simulink model "system_id_new"  (R2023a)
settings: Solver=ode1  StartTime=0.0  StopTime=Sim_time+10  FixedStep=0.002  RelTol=1e-3  EnableMultiTasking=on
values from neighbouring files (symbols this model uses):
  dt = 0.002    [repeated_daqne.m]    (also in test.m)
  frequency = 10.^[f_low:(f_up - f_low)/N_d:f_up-(f_up - f_low)/N_d]'    [repeated_daqne.m]    (also in test.m)
  gain = gain_tuning*rand(size(frequency))    [repeated_daqne.m]    (also in test.m)
  phase = rand(size(frequency))    [repeated_daqne.m]    (also in test.m)
undefined symbols (not defined in the file or in its folder): HIL
libraries: quarc_library x5, slpidlib x1
settings Model: SimulationMode=external  Creator=kentaroohki  LastModifiedBy=Flexible4
settings SolverCC: AlgebraicLoopSolver=TrustRegion  PositivePriorityOrder=on
settings DataIOCC: SaveOperatingPoint=on  SaveFormat=Structure  SaveOutput=off  SignalLogging=off  DSMLogging=off  InspectSignalLogs=on  SaveTime=off  ReturnWorkspaceOutputs=off
settings DebuggingCC: UnconnectedInputMsg=warning  UnconnectedOutputMsg=warning  UnconnectedLineMsg=warning  ArithmeticOperatorsInVariantConditions=warning
settings ModelReferenceCC: EnableRefExpFcnMdlSchedulingChecks=on
settings SFSimCC: SimUseLocalCustomCode=off  CustomCodeUndefinedFunction=UseInterfaceOnly
settings RTWCC: Description=QUARC Win64 Target Using Toolchain  SystemTargetFile=quarc_win64.tlc  TemplateMakefile=quarc_default_tmf  RTWUseLocalCustomCode=off  Toolchain=QUARC win64 | nmake (64-bit Windows)  BuildConfiguration=Faster Runs
settings STFCustomTargetCC: SystemTargetFile=quarc_win64.tlc
settings GRTTargetCC: ParMdlRefBuildCompliant=off  CompOptLevelCompliant=off  CombineOutputUpdateFcns=off  MatFileLogging=off  CPPClassGenCompliant=off  GRTInterface=on  ExtMode=on  ExtModeMexFile=quarc_comm

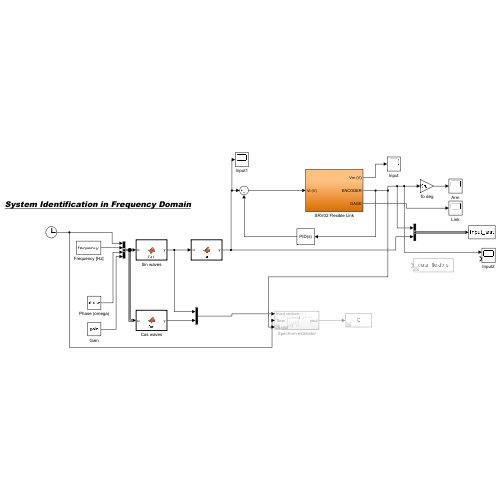
[thumbnail: Simulink's stored preview of the top-level diagram]
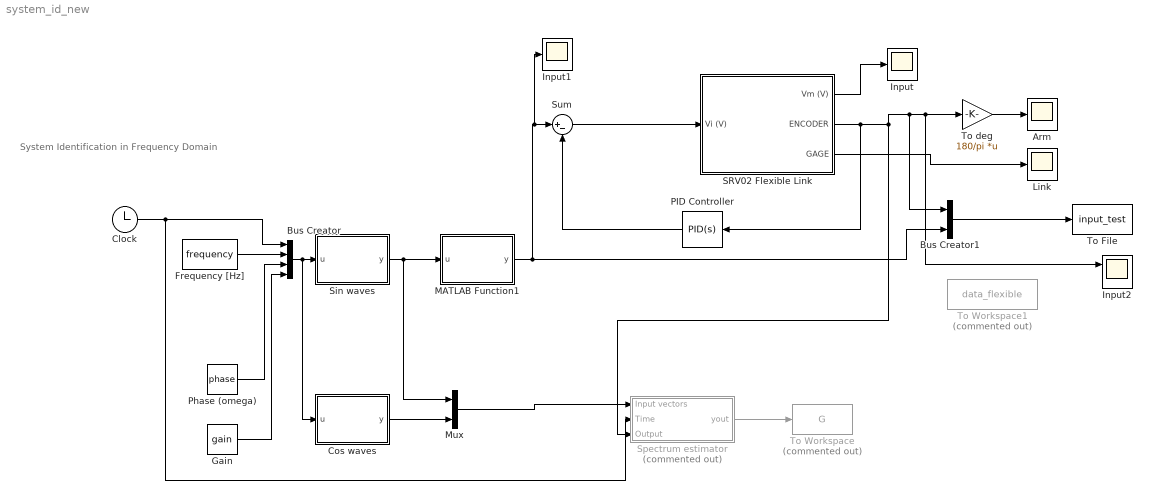
== system system_id_new ==
  note: System Identification in Frequency Domain
  Arm : Scope
  Bus Creator : BusCreator  Inputs=4
  Bus Creator1 : BusCreator  Inputs=2
  Clock : Clock
  Cos waves : MATLAB Function  TreatAsAtomicUnit=on
  Frequency [Hz] : Constant  Value=frequency  VectorParams1D=off
  Gain : Constant  Value=gain  VectorParams1D=off
  Input : Scope
  Input1 : Scope
  Input2 : Scope  NumInputPorts=2
  Link : Scope
  MATLAB Function1 : MATLAB Function  TreatAsAtomicUnit=on
  Mux : Mux  Inputs=2
  PID Controller : slpidlib/PID Controller  Controller=PID  Form=Parallel  TimeDomain=Continuous-time  UseExternalTs=off  SampleTime=-1  IntegratorMethod=Forward Euler  FilterMethod=Forward Euler  ControllerParametersSource=internal  P=1.65  I=0  UseKiTs=off  D=0  N=100  UseFilter=on  TunerSelectOption=Transfer Function Based (PID Tuner App)  InitialConditionSource=internal  InitialConditionForIntegrator=0  InitialConditionForFilter=0  DifferentiatorICPrevScaledInput=0  ExternalReset=none  TrackingMode=off  Kt=1  LimitOutput=off  SatLimitsSource=internal  UpperSaturationLimit=inf  LowerSaturationLimit=-inf  LinearizeAsGain=on  AntiWindupMode=none  Kb=1  LimitIntegrator=off  UpperIntegratorSaturationLimit=inf  LowerIntegratorSaturationLimit=-inf  POutMin=[]  POutMax=[]  IOutMin=[]  IOutMax=[]  DOutMin=[]  DOutMax=[]  NOutMin=[]  NOutMax=[]  SumOutMin=[]  SumOutMax=[]  SaturationOutMin=[]  SaturationOutMax=[]  PParamMin=[]  PParamMax=[]  IParamMin=[]  IParamMax=[]  DParamMin=[]  DParamMax=[]  NParamMin=[]  NParamMax=[]  KbParamMin=[]  KbParamMax=[]  KtParamMin=[]  KtParamMax=[]  KbOutMin=[]  KbOutMax=[]  KtOutMin=[]  KtOutMax=[]  IntegratorOutMin=[]  IntegratorOutMax=[]  FilterOutMin=[]  FilterOutMax=[]  SumI1OutMin=[]  SumI1OutMax=[]  SumI2OutMin=[]  SumI2OutMax=[]  SumI3OutMin=[]  SumI3OutMax=[]  SumI4OutMin=[]  SumI4OutMax=[]  SumDOutMin=[]  SumDOutMax=[]  DifferentiatorOutMin=[]  DifferentiatorOutMax=[]  FilterDiffOutCoefMin=[]  FilterDiffOutCoefMax=[]  ReciprocalOutMin=[]  ReciprocalOutMax=[]  SumDenOutMin=[]  SumDenOutMax=[]  SumNumOutMin=[]  SumNumOutMax=[]  DivideOutMin=[]  DivideOutMax=[]  UdiffTsProdOutMin=[]  UdiffTsProdOutMax=[]  NTsProdOutMin=[]  NTsProdOutMax=[]  UintegralTsProdOutMin=[]  UintegralTsProdOutMax=[]  UngainTsProdOutMin=[]  UngainTsProdOutMax=[]  ClampingZeroOutDataTypeStr=Inherit: Inherit via back propagation  ClampingZeroOutMin=[]  ClampingZeroOutMax=[]  FilterDenConstantOutDataTypeStr=Inherit: Inherit via back propagation  FilterDenConstantOutMin=[]  FilterDenConstantOutMax=[]  PCopyOutDataTypeStr=Inherit: Inherit via back propagation  PCopyOutMin=[]  PCopyOutMax=[]  NCopyOutDataTypeStr=Inherit: Inherit via back propagation  NCopyOutMin=[]  NCopyOutMax=[]  IntegratorContinuousStateAttributes=''  IntegratorStateMustResolveToSignalObject=off  IntegratorRTWStateStorageClass=Auto  FilterContinuousStateAttributes=''  FilterStateMustResolveToSignalObject=off  FilterRTWStateStorageClass=Auto  ParallelPVariant=InternalParameters  IdealPVariant=Disabled  IVariant=InternalParameters  DVariant=InternalParameters  IntegratorVariant=Continuous  SatVariant=Disabled  AWVariant=Passthrough  PCopyVariant=Disabled  TRVariant=Disabled  FdbkBlocksVariant=Forward  IdealPFdbkVariant=Disabled  SatFdbkVariant=Disabled  DerivativeFilterVariant=ContFilter  NVariant=InternalParameters  NCopyVariant=Disabled  FilterICVariant=InternalICsFilter  IntegratorICVariant=InternalICs  ExternalResetVariant=Disabled  TRSumVariant=Passthrough  SumFdbkVariant=Disabled  SumVariant=Sum_PID  TsampFilterVariant=InternalTs  TsampNgainVariant=Passthrough  TsampIntegralVariant=Disabled_SignalSpec  ExternalSaturationOutDataTypeStr=Inherit: Same as second input
  Phase (omega) : Constant  Value=phase  VectorParams1D=off
  SRV02 Flexible Link : Subsystem
  Sin waves : MATLAB Function  TreatAsAtomicUnit=on
  Spectrum estimator : Subsystem  Commented=on
  Sum : Sum  Inputs=|+-
  To File : ToFile  Filename=input_test  MatrixName=output
  To Workspace : ToWorkspace  Commented=on  VariableName=G  SampleTime=dt
      settings: Decimation=decim
  To Workspace1 : ToWorkspace  Commented=on  VariableName=data_flexible  SampleTime=-1
      settings: Save2DSignal=2-D array (concatenate along first dimension)
  To deg : Gain  Gain=180/pi  Multiplication=Matrix(K*u)
  wires:
  SRV02 Flexible Link/3(GAGE) -> Link/1
  Clock/1 -> Spectrum estimator/2(Time), Bus Creator/1
  Frequency [Hz]/1 -> Bus Creator/2
  Phase (omega)/1 -> Bus Creator/3
  Bus Creator/1 -> Cos waves/1(u), Sin waves/1(u)
  Gain/1 -> Bus Creator/4
  Sin waves/1(y) -> Mux/1, MATLAB Function1/1(u)
  MATLAB Function1/1(y) -> Bus Creator1/2, Input1/1, Sum/1
  Spectrum estimator/1(yout) -> To Workspace/1
  Cos waves/1(y) -> Mux/2
  Mux/1 -> Spectrum estimator/1(Input vectors)
  To deg/1 -> Arm/1
  SRV02 Flexible Link/1(Vm (V)) -> Input/1
  SRV02 Flexible Link/2(ENCODER) -> PID Controller/1, Bus Creator1/1, Input2/1, To deg/1, Spectrum estimator/3(Output)
  Sum/1 -> SRV02 Flexible Link/1(Vi (V))
  PID Controller/1 -> Sum/2
  Bus Creator1/1 -> To File/1

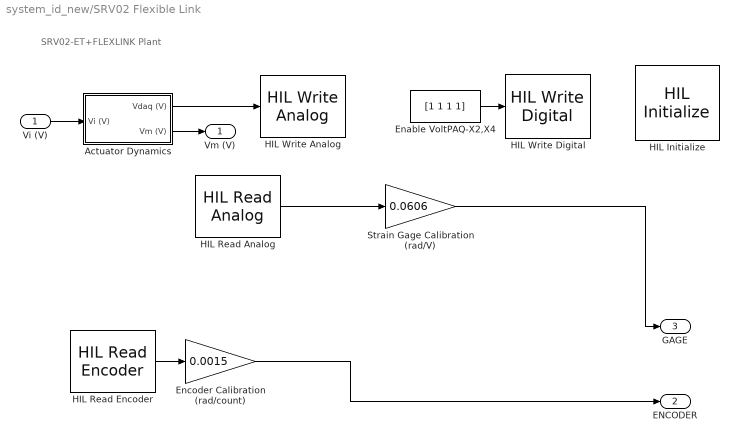
== system system_id_new/SRV02 Flexible Link ==
  note: SRV02-ET+FLEXLINK Plant
  Vi (V) : Inport
  Actuator Dynamics : Subsystem
  Enable VoltPAQ-X2,X4 : Constant  Value=[1 1 1 1]
  Encoder Calibration (rad/count) : Gain  Gain=0.0015  SaturateOnIntegerOverflow=on  OutDataTypeStr=Inherit: Same as input  ParamDataTypeStr=Inherit: Same as input
  HIL Initialize : quarc_library/Data Acquisition/Generic/Configuration/HIL Initialize  object_name=HIL-1  board_type=q2_usb  board_number=0  board_options=d0=digital;d1=digital;led=auto;update_rate=normal  exclusive=off  active=off  hardware_clocks=[0:2]  clock_modes=[]  initial_clock_frequencies=[]  set_clock_params_at_start=off  set_clock_params_at_switch_in=off  set_clock_frequencies_at_start=off  set_clock_frequencies_at_switch_in=off  analog_input_channels=[0:1]  analog_input_configurations=[]  analog_input_maximums=10  analog_input_minimums=-10  set_analog_input_params_at_start=on  set_analog_input_params_at_switch_in=off  analog_output_channels=[0:1]  analog_output_maximums=10  analog_output_minimums=-10  initial_analog_outputs=[0]  final_analog_outputs=[0]  watchdog_analog_outputs=0  set_analog_output_params_at_start=on  set_analog_output_params_at_switch_in=off  set_analog_outputs_at_start=on  set_analog_outputs_at_switch_in=off  set_analog_outputs_at_terminate=on  set_analog_outputs_at_switch_out=off  set_analog_outputs_on_watchdog=off  digital_input_channels=[]  digital_output_channels=[0:7]  digital_output_configuration=[]  initial_digital_outputs=[0]  final_digital_outputs=[0]  watchdog_digital_outputs=[0]  set_digital_output_params_at_start=off  set_digital_output_params_at_switch_in=off  set_digital_outputs_at_start=on  set_digital_outputs_at_switch_in=off  set_digital_outputs_at_terminate=on  set_digital_outputs_at_switch_out=off  set_digital_outputs_on_watchdog=off  encoder_channels=[0:1]  quadrature=[4]  encoder_filter_frequency=[]  initial_encoder_counts=[0]  set_encoder_params_at_start=on  set_encoder_params_at_switch_in=off  set_encoder_counts_at_start=on  set_encoder_counts_at_switch_in=off  pwm_channels=[]  pwm_modes=[0]  pwm_frequency=1/0.020  pwm_configuration=[]  pwm_alignment=[]  pwm_polarity=[]  pwm_leading_deadband=[]  pwm_trailing_deadband=[]  initial_pwm_outputs=[0]  final_pwm_outputs=[0]  watchdog_pwm_outputs=[0]  set_pwm_params_at_start=on  set_pwm_params_at_switch_in=off  set_pwm_outputs_at_start=on  set_pwm_outputs_at_switch_in=off  set_pwm_outputs_at_terminate=on  set_pwm_outputs_at_switch_out=off  set_pwm_outputs_on_watchdog=off  other_output_channels=[]  initial_other_outputs=[]  final_other_outputs=[]  watchdog_other_outputs=[]  set_other_outputs_at_start=off  set_other_outputs_at_switch_in=off  set_other_outputs_at_terminate=off  set_other_outputs_at_switch_out=off  set_other_outputs_on_watchdog=off
  HIL Read Analog : quarc_library/Data Acquisition/Generic/Immediate I//O/HIL Read Analog  object_name=HIL-1  channels=0  sample_time=qc_get_step_size  active=on  vector_output=off
  HIL Read Encoder : quarc_library/Data Acquisition/Generic/Immediate I//O/HIL Read Encoder  object_name=HIL-1  channels=0  sample_time=qc_get_step_size  active=on  vector_output=off  data_type_mode=Inherit via back propagation  data_type=double
  HIL Write Analog : quarc_library/Data Acquisition/Generic/Immediate I//O/HIL Write Analog  object_name=HIL-1  channels=0  sample_time=-1  active=off  vector_input=off
  HIL Write Digital : quarc_library/Data Acquisition/Generic/Immediate I//O/HIL Write Digital  object_name=HIL-1  channels=[0:3]  sample_time=-1  active=off  vector_input=on
      settings: SourceProductName=QUARC Targets
  Strain Gage Calibration (rad/V) : Gain  Gain=0.0606  SaturateOnIntegerOverflow=on  OutDataTypeStr=Inherit: Same as input  ParamDataTypeStr=Inherit: Same as input
  Vm (V) : Outport  InitialOutput=0  VectorParamsAs1DForOutWhenUnconnected=off
  ENCODER : Outport  Port=2  InitialOutput=0  VectorParamsAs1DForOutWhenUnconnected=off
  GAGE : Outport  Port=3  InitialOutput=0  VectorParamsAs1DForOutWhenUnconnected=off
  wires:
  Encoder Calibration (rad/count)/1 -> ENCODER/1
  Actuator Dynamics/2(Vm (V)) -> Vm (V)/1
  Actuator Dynamics/1(Vdaq (V)) -> HIL Write Analog/1
  Vi (V)/1 -> Actuator Dynamics/1(Vi (V))
  Enable VoltPAQ-X2,X4/1 -> HIL Write Digital/1
  HIL Read Analog/1 -> Strain Gage Calibration (rad/V)/1
  Strain Gage Calibration (rad/V)/1 -> GAGE/1
  HIL Read Encoder/1 -> Encoder Calibration (rad/count)/1

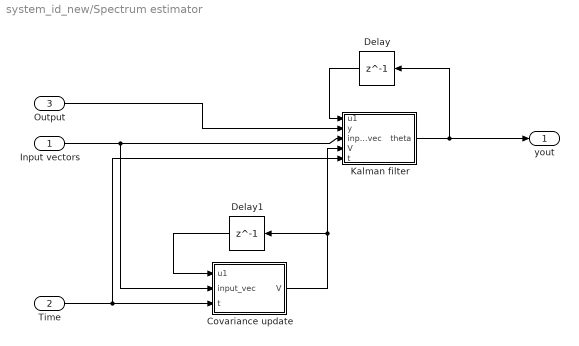
== system system_id_new/Spectrum estimator ==
  Input vectors : Inport
  Time : Inport  Port=2
  Output : Inport  Port=3
  Covariance update : MATLAB Function  TreatAsAtomicUnit=on
  Delay : Delay  DelayLength=1  InitialCondition=0
  Delay1 : Delay  DelayLength=1  InitialCondition=0
  Kalman filter : MATLAB Function  TreatAsAtomicUnit=on
  yout : Outport  VectorParamsAs1DForOutWhenUnconnected=off
  wires:
  Input vectors/1 -> Kalman filter/3(input_vec), Covariance update/2(input_vec)
  Kalman filter/1(theta) -> Delay/1, yout/1
  Delay/1 -> Kalman filter/1(u1)
  Covariance update/1(V) -> Delay1/1, Kalman filter/4(V)
  Delay1/1 -> Covariance update/1(u1)
  Time/1 -> Kalman filter/5(t), Covariance update/3(t)
  Output/1 -> Kalman filter/2(y)

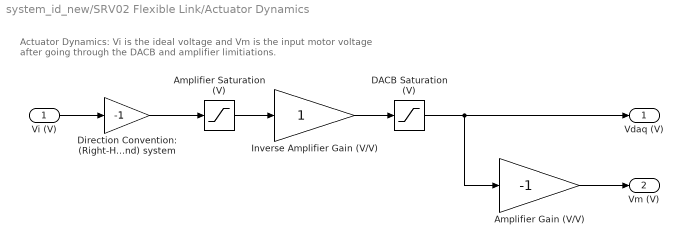
== system system_id_new/SRV02 Flexible Link/Actuator Dynamics ==
  note: Actuator Dynamics: Vi is the ideal voltage and Vm is the
      | input motor voltage after going through the DACB and amplifier limitiations.
  Vi (V) : Inport
  Amplifier Saturation (V) : Saturate  UpperLimit=24  LowerLimit=-24
  Amplifier Gain (V/V) : Gain  Gain=-1
  DACB Saturation (V) : Saturate  UpperLimit=10  LowerLimit=-10
  Direction Convention: (Right-Hand) system : Gain  Gain=-1  SaturateOnIntegerOverflow=on  OutDataTypeStr=Inherit: Same as input  ParamDataTypeStr=Inherit: Same as input
  Inverse Amplifier Gain (V/V) : Gain
  Vdaq (V) : Outport  VectorParamsAs1DForOutWhenUnconnected=off
  Vm (V) : Outport  Port=2  VectorParamsAs1DForOutWhenUnconnected=off
  wires:
  Direction Convention: (Right-Hand) system/1 -> Amplifier Saturation (V)/1
  Amplifier Gain (V/V)/1 -> Vm (V)/1
  DACB Saturation (V)/1 -> Vdaq (V)/1, Amplifier Gain (V/V)/1
  Inverse Amplifier Gain (V/V)/1 -> DACB Saturation (V)/1
  Amplifier Saturation (V)/1 -> Inverse Amplifier Gain (V/V)/1
  Vi (V)/1 -> Direction Convention: (Right-Hand) system/1

== matlab function system_id_new/MATLAB Function1 ==
  data: u input; y output
function y = fcn(u)

 y=sum(u);

== matlab function system_id_new/Sin waves ==
  data: u input; y output
function y = fcn(u)

 n = length(u);% (time) + 3*(#frequencies)
 m = round((n-1)/3);% # of frequencies
 
 y = u(2*m+2:n,1).*sin(2*pi*u(2:m+1,1)*u(1)+u(m+2:2*m+1,1));

== matlab function system_id_new/Spectrum estimator/Kalman filter ==
  data: u1 input; y input; theta output; input_vec input; V input; t input
function theta = fcn(u1,y,input_vec,V,t)

n = length(input_vec);

if t==0.000

    theta = ones(1,n);
else
    theta = u1 - (y + u1*input_vec)/(1+input_vec'*V*input_vec)*input_vec'*V;

end

== matlab function system_id_new/Spectrum estimator/Covariance update ==
  data: u1 input; V output; input_vec input; t input
function V = fcn(u1,input_vec, t)

n = length(input_vec);% 2 * # of frequencies    

if t==0.000
   u1=eye(n,n); 
else
    
    u1 = u1 - u1*input_vec*input_vec'*u1/(1 + input_vec'*u1*input_vec);
    
end
V=u1;

== matlab function system_id_new/Cos waves ==
  data: u input; y output
function y = fcn(u)

 n = length(u);
 m = round((n-1)/3);
 
 y = u(2*m+2:n,1).*cos(2*pi*u(2:m+1,1)*u(1)+u(m+2:2*m+1,1));
